simulink model "ampc_spendulum"  (R2021a)
settings: Solver=ode45  StartTime=0  StopTime=150  MaxStep=0.5*Ts  RelTol=1e-3  EnableMultiTasking=on
values from neighbouring files (symbols this model uses):
  Ts = 0.5    [ampccstr_estimation.m]
  u0 = [op_report.Inputs(1).u;op_report.Inputs(2).u;op_report.Inputs(3).u]    [ampccstr_estimation.m]
  x0 = [op_report.States(1).x;op_report.States(2).x]    [ampccstr_estimation.m]
  y0 = [op_report.Outputs(1).y;op_report.Outputs(2).y]    [ampccstr_estimation.m]
undefined symbols (not defined in the file or in its folder): c, g, l, m
libraries: slident x2, mpclib x1, simulink x1
settings Model: Creator=The MathWorks, Inc.  LastModifiedBy=wmkouw
settings SolverCC: AlgebraicLoopSolver=TrustRegion
settings DataIOCC: ExternalInput=ExtIn  InitialState=[311.267; 8.5695]  SaveFormat=Structure  SaveOutput=off  SignalLogging=off  DSMLogging=off  SaveTime=off  ReturnWorkspaceOutputs=off  SignalLoggingName=logsOut
settings OptimizationCC: BooleanDataType=off  DefaultParameterBehavior=Inlined  InlineInvariantSignals=on  BufferReuse=off  ExpressionDepthLimit=2147483647  InitFltsAndDblsToZero=on  LifeSpan=inf
settings DebuggingCC: SaveWithParameterizedLinksMsg=none  UnderspecifiedInitializationDetection=Classic  MergeDetectMultiDrivingBlocksExec=none  CheckExecutionContextPreStartOutputMsg=on  SignalResolutionControl=TryResolveAllWithWarning  MultiTaskDSMMsg=warning  MultiTaskCondExecSysMsg=none  StateNameClashWarn=warning  SFUnexpectedBacktrackingDiag=warning  SFNoUnconditionalDefaultTransitionDiag=warning  SFExecutionAtInitializationDiag=none  SFMachineParentedDataDiag=warning  ArithmeticOperatorsInVariantConditions=warning
settings HardwareCC: ProdBitPerPointer=32  ProdBitPerSizeT=32  ProdBitPerPtrDiffT=32  ProdLargestAtomicFloat=None  ProdIntDivRoundTo=Undefined  ProdEndianess=Unspecified  ProdWordSize=32  ProdHWDeviceType=32-bit Generic  TargetUnknown=on
settings ModelReferenceCC: PropagateSignalLabelsOutOfModel=off
settings SFSimCC: SimUseLocalCustomCode=off  CustomCodeUndefinedFunction=UseInterfaceOnly
settings RTWCC: RTWUseLocalCustomCode=off
settings CodeAppCC: StateflowObjectComments=on
settings GRTTargetCC: TargetFcnLib=ansi_tfl_tmw.mat  TargetLangStandard=C89/C90 (ANSI)  CombineOutputUpdateFcns=off  GRTInterface=on
settings ConfigComp: CovMetricSettings=dw  CovSaveCumulativeToWorkspaceVar=on  CovSaveSingleToWorkspaceVar=on  CovExternalEMLEnable=off  CovSFcnEnable=off

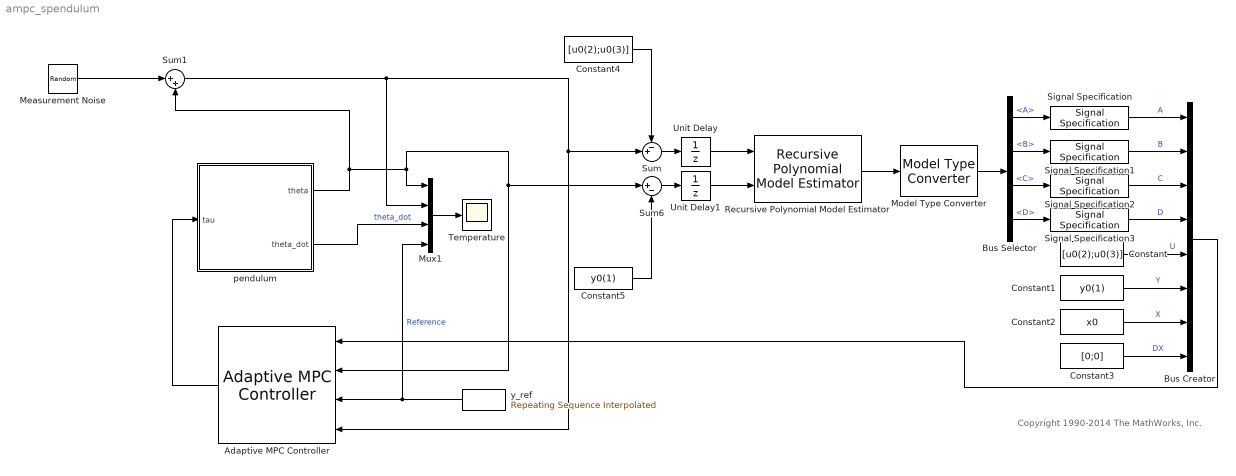
== system ampc_spendulum ==
  note: Copyright 1990-2014 The MathWorks, Inc.
  Adaptive MPC Controller : mpclib/Adaptive MPC Controller  SCDEnableBlockLinearizationSpecification=on  mpcobj=mpcobj  enable_value=0  updateMPCinCallerWorkspace=on  md_inport=on  mv_inport=off  uref_inport=off  return_cost=off  return_mvseq=off  return_qpstatus=off  return_xseq=off  return_state=off  return_ovseq=off  state_inport=off  isltv_plant=off  umin_inport=off  umax_inport=off  ymin_inport=off  ymax_inport=off  cc_inport=off  ywt_inport=off  uwt_inport=off  duwt_inport=off  rhoeps_inport=off  pm_inport=off  MaximumP=10  HorizonChoice=FixedHorizon  BlockDataType=double  SampleTimeInherited=off  switch_inport=off
  Bus Creator : BusCreator  Inputs=8
  Bus Selector : BusSelector  OutputSignals=A,B,C,D
  Constant : Constant  Value=[u0(2);u0(3)]  VectorParams1D=off
  Constant1 : Constant  Value=y0(1)  VectorParams1D=off
  Constant2 : Constant  Value=x0  VectorParams1D=off
  Constant3 : Constant  Value=[0;0]  VectorParams1D=off
  Constant4 : Constant  Value=[u0(2);u0(3)]
  Constant5 : Constant  Value=y0(1)
  Measurement Noise : RandomNumber  Variance=0.01  Seed=12345  SampleTime=Ts
  Model Type Converter : slident/Estimators/Model Type Converter  InputModelType=ARX
      settings: SourceProductBaseCode=ID
  Mux1 : Mux
  Recursive Polynomial Model Estimator : slident/Estimators/Recursive Polynomial Model Estimator  ModelStructure=ARX  InitialEstimateSource=Internal  A0=Aq  B0=Bq  C0=1  D0=1  F0=1  nk=1  P0=1  InitialInputs=0  InitialOutputs=0  History=Infinite  WindowLength=200  EstimationMethod=Kalman Filter  AdaptationParameter=0.01  HasTimeVaryingAdaptationParameter=off  NormalizationBias=eps  OutputError=off  OutputP=off  AddEnablePort=off  InputProcessing=Sample-based  Ts=Ts
      settings: SourceProductBaseCode=ID
  Signal Specification : SignalSpecification  Dimensions=[2 2]
  Signal Specification1 : SignalSpecification  Dimensions=[2 2]
  Signal Specification2 : SignalSpecification  Dimensions=[1 2]
  Signal Specification3 : SignalSpecification  Dimensions=[1 2]
  Sum : Sum  Inputs=-+|
  Sum1 : Sum  Inputs=|++  SampleTime=Ts
  Sum6 : Sum  Inputs=|+-
  Temperature : Scope
  Unit Delay : UnitDelay  InitialCondition=[0;0]  SampleTime=Ts  HasFrameUpgradeWarning=on
  Unit Delay1 : UnitDelay  SampleTime=Ts  HasFrameUpgradeWarning=on
  pendulum : Subsystem
  y_ref : simulink/Sources/Repeating Sequence Interpolated  OutValues=y_ref  TimeValues=0  LookUpMeth=Interpolation-Use End Values  tsamp=Ts  OutMin=[]  OutMax=[]  OutDataTypeStr=double  OutputDataTypeScalingMode=double  OutDataType=fixdt(0,8)  OutScaling=2^-10
  wires:
  Mux1/1 -> Temperature/1
  Sum1/1 -> Sum/2, Adaptive MPC Controller/4, Mux1/2
  Bus Creator/1 -> Adaptive MPC Controller/1
  pendulum/1(theta) -> Adaptive MPC Controller/2, Sum6/1, Mux1/1, Sum1/2
  y_ref/1 -> Adaptive MPC Controller/3, Mux1/4  "Reference"
  Measurement Noise/1 -> Sum1/1
  Unit Delay1/1 -> Recursive Polynomial Model Estimator/2
  Model Type Converter/1 -> Bus Selector/1
  Recursive Polynomial Model Estimator/1 -> Model Type Converter/1
  Constant1/1 -> Bus Creator/6  "Y"
  Constant/1 -> Bus Creator/5  "U"
  Bus Selector/1 -> Signal Specification/1  "<A>"
  Signal Specification/1 -> Bus Creator/1  "A"
  Bus Selector/2 -> Signal Specification1/1  "<B>"
  Bus Selector/3 -> Signal Specification2/1  "<C>"
  Bus Selector/4 -> Signal Specification3/1  "<D>"
  Signal Specification1/1 -> Bus Creator/2  "B"
  Signal Specification2/1 -> Bus Creator/3  "C"
  Signal Specification3/1 -> Bus Creator/4  "D"
  Constant2/1 -> Bus Creator/7  "X"
  Constant3/1 -> Bus Creator/8  "DX"
  Adaptive MPC Controller/1 -> pendulum/1(tau)
  Sum6/1 -> Unit Delay1/1
  Sum/1 -> Unit Delay/1
  Constant4/1 -> Sum/1
  Unit Delay/1 -> Recursive Polynomial Model Estimator/1
  Constant5/1 -> Sum6/2
  pendulum/2(theta_dot) -> Mux1/3  "theta_dot"

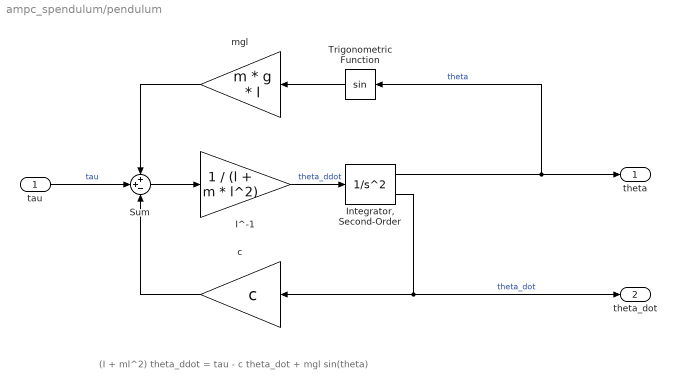
== system ampc_spendulum/pendulum ==
  note: (I + ml^2) theta_ddot = tau - c theta_dot + mgl sin(theta)
  tau : Inport
  I^-1 : Gain  Gain=1 / (l + m * l^2)
  "Integrator, Second-Order" : SecondOrderIntegrator  ICX=theta0  UpperLimitX=1  LowerLimitX=0  StateNameX='theta'  ICDXDT=theta_dot0  StateNameDXDT='theta_dot'
  Sum : Sum  Inputs=++-
  Trigonometric Function : Trigonometry
  c : Gain  Gain=c
  mgl : Gain  Gain=m * g * l
  theta : Outport  VectorParamsAs1DForOutWhenUnconnected=off
  theta_dot : Outport  Port=2  VectorParamsAs1DForOutWhenUnconnected=off
  wires:
  mgl/1 -> Sum/1
  c/1 -> Sum/3
  Trigonometric Function/1 -> mgl/1
  Sum/1 -> I^-1/1
  "Integrator, Second-Order"/1 -> theta/1, Trigonometric Function/1  "theta"
  I^-1/1 -> "Integrator, Second-Order"/1  "theta_ddot"
  "Integrator, Second-Order"/2 -> c/1, theta_dot/1  "theta_dot"
  tau/1 -> Sum/2  "tau"
